simulink model "Dianlan_deng"  (R2021a)
settings: Solver=ode23tb  StartTime=0.0  StopTime=20e-6  MaxStep=0.2  RelTol=1e-4  EnableMultiTasking=on
PreLoadFcn:
  | % -- Recommended Settings --
  | %
  | %  Simulink:
  | %      Solver: Ode23tb
  | %      Relative tolerance = 1e-4
  | %      Max step size = 0.2
  | %
  | %  Powergui:
  |          Ts = 0; % (continuous electrical model)
  | %
  | %
  | % ----------------------------------
libraries: spsVoltageMeasurementLib x4, spsDistributedParametersLineLib x3, spsGroundLib x3, spsSeriesRLCBranchLib x3, spsControlledVoltageSourceLib x1, spspowerguiLib x1
settings Model: Creator=Administrator  LastModifiedBy=张瑞
settings SolverCC: AlgebraicLoopSolver=TrustRegion
settings DataIOCC: LimitDataPoints=on  ReturnWorkspaceOutputs=off
settings OptimizationCC: LifeSpan=inf
settings DebuggingCC: AllowSymbolicDim=off  SFUnexpectedBacktrackingDiag=warning  SFNoUnconditionalDefaultTransitionDiag=warning  SFMachineParentedDataDiag=warning  ArithmeticOperatorsInVariantConditions=warning
settings SFSimCC: SimUseLocalCustomCode=off  CustomCodeUndefinedFunction=UseInterfaceOnly
settings RTWCC: RTWUseLocalCustomCode=off
settings CodeAppCC: StateflowObjectComments=on
settings GRTTargetCC: TargetLangStandard=C89/C90 (ANSI)
settings ConfigComp: CovMetricSettings=dw  CovSaveCumulativeToWorkspaceVar=on  CovSaveSingleToWorkspaceVar=on  CovExternalEMLEnable=off  CovSFcnEnable=off
settings SimscapeCC: SimscapeNormalizeSystem=off

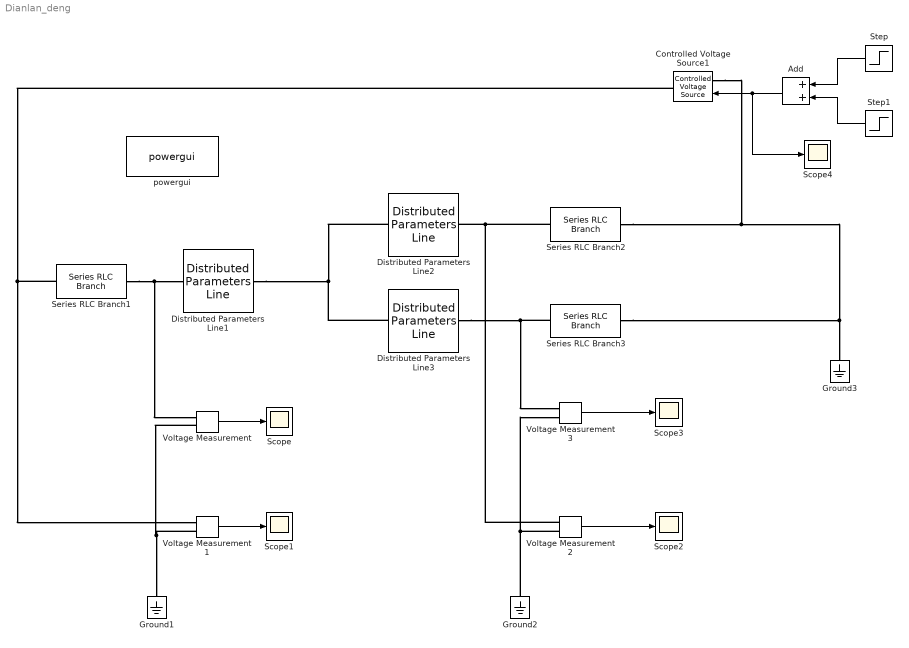
== system Dianlan_deng ==
  Add : Sum
  Controlled Voltage Source1 : spsControlledVoltageSourceLib/Controlled Voltage Source  Initialize=off  Source_Type=DC  Amplitude=0  Phase=0  Frequency=0  Measurements=Voltage
  Distributed Parameters Line1 : spsDistributedParametersLineLib/Distributed Parameters Line  Phases=1  Length=0.2  Frequency=1000  Resistance=1.8E-1  Inductance=2.75E-4  Capacitance=5.57E-7  x1=[-2.48e-06 0;-2.47e-06 0;-2.46e-06 0;-2.45e-06 0;-2.44e-06 0;-2.43e-06 0;-2.42e-06 0;-2.41e-06 0;-2.4e-06 0;-2.39e-06 0;-2.38e-06 0;-2.37e-06 0;-2.36e-06 0;-2.35e-06 0;-2.34e-06 0;-2.33e-06 0;-2.32e-06 0;-2.31e-06 0;-2.3e-06 0;-2.29e-06 0;-2.28e-06 0;-2.27e-06 0;-2.26e-06 0;-2.25e-06 0;-2.24e-06 0;-2.23e-06 0;-2.22e-06 0;-2.21e-06 0;-2.2e-06 0;-2.19e-06 0;-2.18e-06 0;-2.17e-06 0;-2.16e-06 0;-2.15e-06 0;-2.14e-06 0;-2.13e-06 0;-2.12e-06 0;-2.11e-06 0;-2.1e-06 0;-2.09e-06 0;-2.08e-06 0;-2.07e-06 0;-2.06e-06 0;-2.05e-06 0;-2.04e-06 0;-2.03e-06 0;-2.02e-06 0;-2.01e-06 0;-2e-06 0;-1.99e-06 0;-1.98e-06 0;-1.97e-06 0;-1.96e-06 0;-1.95e-06 0;-1.94e-06 0;-1.93e-06 0;-1.92e-06 0;-1.91e-06 0;-1.9e-06 0;-1.89e-06 0;-1.88e-06 0;-1.87e-06 0;-1.86e-06 0;-1.85e-06 0;-1.84e-06 0;-1.83e-06 0;-1.82e-06 0;-1.81e-06 0;-1.8e-06 0;-1.79e-06 0;-1.78e-06 0;-1.77e-06 0;-1.76e-06 0;-1.75e-06 0;-1.74e-06 0;-1.73e-06 0;-1.72e-06 0;-1.71e-06 0;-1.7e-06 0;-1.69e-06 0;-1.68e-06 0;-1.67e-06 0;-1.66e-06 0;-1.65e-06 0;-1.64e-06 0;-1.63e-06 0;-1.62e-06 0;-1.61e-06 0;-1.6e-06 0;-1.59e-06 0;-1.58e-06 0;-1.57e-06 0;-1.56e-06 0;-1.55e-06 0;-1.54e-06 0;-1.53e-06 0;-1.52e-06 0;-1.51e-06 0;-1.5e-06 0;-1.49e-06 0;-1.48e-06 0;-1.47e-06 0;-1.46e-06 0;-1.45e-06 0;-1.44e-06 0;-1.43e-06 0;-1.42e-06 0;-1.41e-06 0;-1.4e-06 0;-1.39e-06 0;-1.38e-06 0;-1.37e-06 0;-1.36e-06 0;-1.35e-06 0;-1.34e-06 0;-1.33e-06 0;-1.32e-06 0;-1.31e-06 0;-1.3e-06 0;-1.29e-06 0;-1.28e-06 0;-1.27e-06 0;-1.26e-06 0;-1.25e-06 0;-1.24e-06 0;-1.23e-06 0;-1.22e-06 0;-1.21e-06 0;-1.2e-06 0;-1.19e-06 0;-1.18e-06 0;-1.17e-06 0;-1.16e-06 0;-1.15e-06 0;-1.14e-06 0;-1.13e-06 0;-1.12e-06 0;-1.11e-06 0;-1.1e-06 0;-1.09e-06 0;-1.08e-06 0;-1.07e-06 0;-1.06e-06 0;-1.05e-06 0;-1.04e-06 0;-1.03e-06 0;-1.02e-06 0;-1.01e-06 0;-1e-06 0;-9.9e-07 0;-9.8e-07 0;-9.7e-07 0;-9.6e-07 0;-9.5e-07 0;-9.4e-07 0;-9.3e-07 0;-9.2e-07 0;-9.1e-07 0;-9e-07 0;-8.9e-07 0;-8.8e-07 0;-8.7e-07 0;-8.6e-07 0;-8.5e-07 0;-8.4e-07 0;-8.3e-07 0;-8.2e-07 0;-8.1e-07 0;-8e-07 0;-7.9e-07 0;-7.8e-07 0;-7.7e-07 0;-7.6e-07 0;-7.5e-07 0;-7.4e-07 0;-7.3e-07 0;-7.2e-07 0;-7.1e-07 0;-7e-07 0;-6.9e-07 0;-6.8e-07 0;-6.7e-07 0;-6.6e-07 0;-6.5e-07 0;-6.4e-07 0;-6.3e-07 0;-6.2e-07 0;-6.1e-07 0;-6e-07 0;-5.9e-07 0;-5.8e-07 0;-5.7e-07 0;-5.6e-07 0;-5.5e-07 0;-5.4e-07 0;-5.3e-07 0;-5.2e-07 0;-5.1e-07 0;-5e-07 0;-4.9e-07 0;-4.8e-07 0;-4.7e-07 0;-4.6e-07 0;-4.5e-07 0;-4.4e-07 0;-4.3e-07 0;-4.2e-07 0;-4.1e-07 0;-4e-07 0;-3.9e-07 0;-3.8e-07 0;-3.7e-07 0;-3.6e-07 0;-3.5e-07 0;-3.4e-07 0;-3.3e-07 0;-3.2e-07 0;-3.1e-07 0;-3e-07 0;-2.9e-07 0;-2.8e-07 0;-2.7e-07 0;-2.6e-07 0;-2.5e-07 0;-2.4e-07 0;-2.3e-07 0;-2.2e-07 0;-2.1e-07 0;-2e-07 0;-1.9e-07 0;-1.8e-07 0;-1.7e-07 0;-1.6e-07 0;-1.5e-07 0;-1.4e-07 0;-1.3e-07 0;-1.2e-07 0;-1.1e-07 0;-1e-07 0;-9e-08 0;-8e-08 0;-7e-08 0;-6e-08 0;-5e-08 0;-4e-08 0;-3e-08 0;-2e-08 0;-1e-08 0]  x2=[-2.48e-06 0;-2.47e-06 0;-2.46e-06 0;-2.45e-06 0;-2.44e-06 0;-2.43e-06 0;-2.42e-06 0;-2.41e-06 0;-2.4e-06 0;-2.39e-06 0;-2.38e-06 0;-2.37e-06 0;-2.36e-06 0;-2.35e-06 0;-2.34e-06 0;-2.33e-06 0;-2.32e-06 0;-2.31e-06 0;-2.3e-06 0;-2.29e-06 0;-2.28e-06 0;-2.27e-06 0;-2.26e-06 0;-2.25e-06 0;-2.24e-06 0;-2.23e-06 0;-2.22e-06 0;-2.21e-06 0;-2.2e-06 0;-2.19e-06 0;-2.18e-06 0;-2.17e-06 0;-2.16e-06 0;-2.15e-06 0;-2.14e-06 0;-2.13e-06 0;-2.12e-06 0;-2.11e-06 0;-2.1e-06 0;-2.09e-06 0;-2.08e-06 0;-2.07e-06 0;-2.06e-06 0;-2.05e-06 0;-2.04e-06 0;-2.03e-06 0;-2.02e-06 0;-2.01e-06 0;-2e-06 0;-1.99e-06 0;-1.98e-06 0;-1.97e-06 0;-1.96e-06 0;-1.95e-06 0;-1.94e-06 0;-1.93e-06 0;-1.92e-06 0;-1.91e-06 0;-1.9e-06 0;-1.89e-06 0;-1.88e-06 0;-1.87e-06 0;-1.86e-06 0;-1.85e-06 0;-1.84e-06 0;-1.83e-06 0;-1.82e-06 0;-1.81e-06 0;-1.8e-06 0;-1.79e-06 0;-1.78e-06 0;-1.77e-06 0;-1.76e-06 0;-1.75e-06 0;-1.74e-06 0;-1.73e-06 0;-1.72e-06 0;-1.71e-06 0;-1.7e-06 0;-1.69e-06 0;-1.68e-06 0;-1.67e-06 0;-1.66e-06 0;-1.65e-06 0;-1.64e-06 0;-1.63e-06 0;-1.62e-06 0;-1.61e-06 0;-1.6e-06 0;-1.59e-06 0;-1.58e-06 0;-1.57e-06 0;-1.56e-06 0;-1.55e-06 0;-1.54e-06 0;-1.53e-06 0;-1.52e-06 0;-1.51e-06 0;-1.5e-06 0;-1.49e-06 0;-1.48e-06 0;-1.47e-06 0;-1.46e-06 0;-1.45e-06 0;-1.44e-06 0;-1.43e-06 0;-1.42e-06 0;-1.41e-06 0;-1.4e-06 0;-1.39e-06 0;-1.38e-06 0;-1.37e-06 0;-1.36e-06 0;-1.35e-06 0;-1.34e-06 0;-1.33e-06 0;-1.32e-06 0;-1.31e-06 0;-1.3e-06 0;-1.29e-06 0;-1.28e-06 0;-1.27e-06 0;-1.26e-06 0;-1.25e-06 0;-1.24e-06 0;-1.23e-06 0;-1.22e-06 0;-1.21e-06 0;-1.2e-06 0;-1.19e-06 0;-1.18e-06 0;-1.17e-06 0;-1.16e-06 0;-1.15e-06 0;-1.14e-06 0;-1.13e-06 0;-1.12e-06 0;-1.11e-06 0;-1.1e-06 0;-1.09e-06 0;-1.08e-06 0;-1.07e-06 0;-1.06e-06 0;-1.05e-06 0;-1.04e-06 0;-1.03e-06 0;-1.02e-06 0;-1.01e-06 0;-1e-06 0;-9.9e-07 0;-9.8e-07 0;-9.7e-07 0;-9.6e-07 0;-9.5e-07 0;-9.4e-07 0;-9.3e-07 0;-9.2e-07 0;-9.1e-07 0;-9e-07 0;-8.9e-07 0;-8.8e-07 0;-8.7e-07 0;-8.6e-07 0;-8.5e-07 0;-8.4e-07 0;-8.3e-07 0;-8.2e-07 0;-8.1e-07 0;-8e-07 0;-7.9e-07 0;-7.8e-07 0;-7.7e-07 0;-7.6e-07 0;-7.5e-07 0;-7.4e-07 0;-7.3e-07 0;-7.2e-07 0;-7.1e-07 0;-7e-07 0;-6.9e-07 0;-6.8e-07 0;-6.7e-07 0;-6.6e-07 0;-6.5e-07 0;-6.4e-07 0;-6.3e-07 0;-6.2e-07 0;-6.1e-07 0;-6e-07 0;-5.9e-07 0;-5.8e-07 0;-5.7e-07 0;-5.6e-07 0;-5.5e-07 0;-5.4e-07 0;-5.3e-07 0;-5.2e-07 0;-5.1e-07 0;-5e-07 0;-4.9e-07 0;-4.8e-07 0;-4.7e-07 0;-4.6e-07 0;-4.5e-07 0;-4.4e-07 0;-4.3e-07 0;-4.2e-07 0;-4.1e-07 0;-4e-07 0;-3.9e-07 0;-3.8e-07 0;-3.7e-07 0;-3.6e-07 0;-3.5e-07 0;-3.4e-07 0;-3.3e-07 0;-3.2e-07 0;-3.1e-07 0;-3e-07 0;-2.9e-07 0;-2.8e-07 0;-2.7e-07 0;-2.6e-07 0;-2.5e-07 0;-2.4e-07 0;-2.3e-07 0;-2.2e-07 0;-2.1e-07 0;-2e-07 0;-1.9e-07 0;-1.8e-07 0;-1.7e-07 0;-1.6e-07 0;-1.5e-07 0;-1.4e-07 0;-1.3e-07 0;-1.2e-07 0;-1.1e-07 0;-1e-07 0;-9e-08 0;-8e-08 0;-7e-08 0;-6e-08 0;-5e-08 0;-4e-08 0;-3e-08 0;-2e-08 0;-1e-08 0]  x3=[-2.48e-06 0;-2.47e-06 0;-2.46e-06 0;-2.45e-06 0;-2.44e-06 0;-2.43e-06 0;-2.42e-06 0;-2.41e-06 0;-2.4e-06 0;-2.39e-06 0;-2.38e-06 0;-2.37e-06 0;-2.36e-06 0;-2.35e-06 0;-2.34e-06 0;-2.33e-06 0;-2.32e-06 0;-2.31e-06 0;-2.3e-06 0;-2.29e-06 0;-2.28e-06 0;-2.27e-06 0;-2.26e-06 0;-2.25e-06 0;-2.24e-06 0;-2.23e-06 0;-2.22e-06 0;-2.21e-06 0;-2.2e-06 0;-2.19e-06 0;-2.18e-06 0;-2.17e-06 0;-2.16e-06 0;-2.15e-06 0;-2.14e-06 0;-2.13e-06 0;-2.12e-06 0;-2.11e-06 0;-2.1e-06 0;-2.09e-06 0;-2.08e-06 0;-2.07e-06 0;-2.06e-06 0;-2.05e-06 0;-2.04e-06 0;-2.03e-06 0;-2.02e-06 0;-2.01e-06 0;-2e-06 0;-1.99e-06 0;-1.98e-06 0;-1.97e-06 0;-1.96e-06 0;-1.95e-06 0;-1.94e-06 0;-1.93e-06 0;-1.92e-06 0;-1.91e-06 0;-1.9e-06 0;-1.89e-06 0;-1.88e-06 0;-1.87e-06 0;-1.86e-06 0;-1.85e-06 0;-1.84e-06 0;-1.83e-06 0;-1.82e-06 0;-1.81e-06 0;-1.8e-06 0;-1.79e-06 0;-1.78e-06 0;-1.77e-06 0;-1.76e-06 0;-1.75e-06 0;-1.74e-06 0;-1.73e-06 0;-1.72e-06 0;-1.71e-06 0;-1.7e-06 0;-1.69e-06 0;-1.68e-06 0;-1.67e-06 0;-1.66e-06 0;-1.65e-06 0;-1.64e-06 0;-1.63e-06 0;-1.62e-06 0;-1.61e-06 0;-1.6e-06 0;-1.59e-06 0;-1.58e-06 0;-1.57e-06 0;-1.56e-06 0;-1.55e-06 0;-1.54e-06 0;-1.53e-06 0;-1.52e-06 0;-1.51e-06 0;-1.5e-06 0;-1.49e-06 0;-1.48e-06 0;-1.47e-06 0;-1.46e-06 0;-1.45e-06 0;-1.44e-06 0;-1.43e-06 0;-1.42e-06 0;-1.41e-06 0;-1.4e-06 0;-1.39e-06 0;-1.38e-06 0;-1.37e-06 0;-1.36e-06 0;-1.35e-06 0;-1.34e-06 0;-1.33e-06 0;-1.32e-06 0;-1.31e-06 0;-1.3e-06 0;-1.29e-06 0;-1.28e-06 0;-1.27e-06 0;-1.26e-06 0;-1.25e-06 0;-1.24e-06 0;-1.23e-06 0;-1.22e-06 0;-1.21e-06 0;-1.2e-06 0;-1.19e-06 0;-1.18e-06 0;-1.17e-06 0;-1.16e-06 0;-1.15e-06 0;-1.14e-06 0;-1.13e-06 0;-1.12e-06 0;-1.11e-06 0;-1.1e-06 0;-1.09e-06 0;-1.08e-06 0;-1.07e-06 0;-1.06e-06 0;-1.05e-06 0;-1.04e-06 0;-1.03e-06 0;-1.02e-06 0;-1.01e-06 0;-1e-06 0;-9.9e-07 0;-9.8e-07 0;-9.7e-07 0;-9.6e-07 0;-9.5e-07 0;-9.4e-07 0;-9.3e-07 0;-9.2e-07 0;-9.1e-07 0;-9e-07 0;-8.9e-07 0;-8.8e-07 0;-8.7e-07 0;-8.6e-07 0;-8.5e-07 0;-8.4e-07 0;-8.3e-07 0;-8.2e-07 0;-8.1e-07 0;-8e-07 0;-7.9e-07 0;-7.8e-07 0;-7.7e-07 0;-7.6e-07 0;-7.5e-07 0;-7.4e-07 0;-7.3e-07 0;-7.2e-07 0;-7.1e-07 0;-7e-07 0;-6.9e-07 0;-6.8e-07 0;-6.7e-07 0;-6.6e-07 0;-6.5e-07 0;-6.4e-07 0;-6.3e-07 0;-6.2e-07 0;-6.1e-07 0;-6e-07 0;-5.9e-07 0;-5.8e-07 0;-5.7e-07 0;-5.6e-07 0;-5.5e-07 0;-5.4e-07 0;-5.3e-07 0;-5.2e-07 0;-5.1e-07 0;-5e-07 0;-4.9e-07 0;-4.8e-07 0;-4.7e-07 0;-4.6e-07 0;-4.5e-07 0;-4.4e-07 0;-4.3e-07 0;-4.2e-07 0;-4.1e-07 0;-4e-07 0;-3.9e-07 0;-3.8e-07 0;-3.7e-07 0;-3.6e-07 0;-3.5e-07 0;-3.4e-07 0;-3.3e-07 0;-3.2e-07 0;-3.1e-07 0;-3e-07 0;-2.9e-07 0;-2.8e-07 0;-2.7e-07 0;-2.6e-07 0;-2.5e-07 0;-2.4e-07 0;-2.3e-07 0;-2.2e-07 0;-2.1e-07 0;-2e-07 0;-1.9e-07 0;-1.8e-07 0;-1.7e-07 0;-1.6e-07 0;-1.5e-07 0;-1.4e-07 0;-1.3e-07 0;-1.2e-07 0;-1.1e-07 0;-1e-07 0;-9e-08 0;-8e-08 0;-7e-08 0;-6e-08 0;-5e-08 0;-4e-08 0;-3e-08 0;-2e-08 0;-1e-08 0]  x4=[-2.48e-06 0;-2.47e-06 0;-2.46e-06 0;-2.45e-06 0;-2.44e-06 0;-2.43e-06 0;-2.42e-06 0;-2.41e-06 0;-2.4e-06 0;-2.39e-06 0;-2.38e-06 0;-2.37e-06 0;-2.36e-06 0;-2.35e-06 0;-2.34e-06 0;-2.33e-06 0;-2.32e-06 0;-2.31e-06 0;-2.3e-06 0;-2.29e-06 0;-2.28e-06 0;-2.27e-06 0;-2.26e-06 0;-2.25e-06 0;-2.24e-06 0;-2.23e-06 0;-2.22e-06 0;-2.21e-06 0;-2.2e-06 0;-2.19e-06 0;-2.18e-06 0;-2.17e-06 0;-2.16e-06 0;-2.15e-06 0;-2.14e-06 0;-2.13e-06 0;-2.12e-06 0;-2.11e-06 0;-2.1e-06 0;-2.09e-06 0;-2.08e-06 0;-2.07e-06 0;-2.06e-06 0;-2.05e-06 0;-2.04e-06 0;-2.03e-06 0;-2.02e-06 0;-2.01e-06 0;-2e-06 0;-1.99e-06 0;-1.98e-06 0;-1.97e-06 0;-1.96e-06 0;-1.95e-06 0;-1.94e-06 0;-1.93e-06 0;-1.92e-06 0;-1.91e-06 0;-1.9e-06 0;-1.89e-06 0;-1.88e-06 0;-1.87e-06 0;-1.86e-06 0;-1.85e-06 0;-1.84e-06 0;-1.83e-06 0;-1.82e-06 0;-1.81e-06 0;-1.8e-06 0;-1.79e-06 0;-1.78e-06 0;-1.77e-06 0;-1.76e-06 0;-1.75e-06 0;-1.74e-06 0;-1.73e-06 0;-1.72e-06 0;-1.71e-06 0;-1.7e-06 0;-1.69e-06 0;-1.68e-06 0;-1.67e-06 0;-1.66e-06 0;-1.65e-06 0;-1.64e-06 0;-1.63e-06 0;-1.62e-06 0;-1.61e-06 0;-1.6e-06 0;-1.59e-06 0;-1.58e-06 0;-1.57e-06 0;-1.56e-06 0;-1.55e-06 0;-1.54e-06 0;-1.53e-06 0;-1.52e-06 0;-1.51e-06 0;-1.5e-06 0;-1.49e-06 0;-1.48e-06 0;-1.47e-06 0;-1.46e-06 0;-1.45e-06 0;-1.44e-06 0;-1.43e-06 0;-1.42e-06 0;-1.41e-06 0;-1.4e-06 0;-1.39e-06 0;-1.38e-06 0;-1.37e-06 0;-1.36e-06 0;-1.35e-06 0;-1.34e-06 0;-1.33e-06 0;-1.32e-06 0;-1.31e-06 0;-1.3e-06 0;-1.29e-06 0;-1.28e-06 0;-1.27e-06 0;-1.26e-06 0;-1.25e-06 0;-1.24e-06 0;-1.23e-06 0;-1.22e-06 0;-1.21e-06 0;-1.2e-06 0;-1.19e-06 0;-1.18e-06 0;-1.17e-06 0;-1.16e-06 0;-1.15e-06 0;-1.14e-06 0;-1.13e-06 0;-1.12e-06 0;-1.11e-06 0;-1.1e-06 0;-1.09e-06 0;-1.08e-06 0;-1.07e-06 0;-1.06e-06 0;-1.05e-06 0;-1.04e-06 0;-1.03e-06 0;-1.02e-06 0;-1.01e-06 0;-1e-06 0;-9.9e-07 0;-9.8e-07 0;-9.7e-07 0;-9.6e-07 0;-9.5e-07 0;-9.4e-07 0;-9.3e-07 0;-9.2e-07 0;-9.1e-07 0;-9e-07 0;-8.9e-07 0;-8.8e-07 0;-8.7e-07 0;-8.6e-07 0;-8.5e-07 0;-8.4e-07 0;-8.3e-07 0;-8.2e-07 0;-8.1e-07 0;-8e-07 0;-7.9e-07 0;-7.8e-07 0;-7.7e-07 0;-7.6e-07 0;-7.5e-07 0;-7.4e-07 0;-7.3e-07 0;-7.2e-07 0;-7.1e-07 0;-7e-07 0;-6.9e-07 0;-6.8e-07 0;-6.7e-07 0;-6.6e-07 0;-6.5e-07 0;-6.4e-07 0;-6.3e-07 0;-6.2e-07 0;-6.1e-07 0;-6e-07 0;-5.9e-07 0;-5.8e-07 0;-5.7e-07 0;-5.6e-07 0;-5.5e-07 0;-5.4e-07 0;-5.3e-07 0;-5.2e-07 0;-5.1e-07 0;-5e-07 0;-4.9e-07 0;-4.8e-07 0;-4.7e-07 0;-4.6e-07 0;-4.5e-07 0;-4.4e-07 0;-4.3e-07 0;-4.2e-07 0;-4.1e-07 0;-4e-07 0;-3.9e-07 0;-3.8e-07 0;-3.7e-07 0;-3.6e-07 0;-3.5e-07 0;-3.4e-07 0;-3.3e-07 0;-3.2e-07 0;-3.1e-07 0;-3e-07 0;-2.9e-07 0;-2.8e-07 0;-2.7e-07 0;-2.6e-07 0;-2.5e-07 0;-2.4e-07 0;-2.3e-07 0;-2.2e-07 0;-2.1e-07 0;-2e-07 0;-1.9e-07 0;-1.8e-07 0;-1.7e-07 0;-1.6e-07 0;-1.5e-07 0;-1.4e-07 0;-1.3e-07 0;-1.2e-07 0;-1.1e-07 0;-1e-07 0;-9e-08 0;-8e-08 0;-7e-08 0;-6e-08 0;-5e-08 0;-4e-08 0;-3e-08 0;-2e-08 0;-1e-08 0]  x5=2.47527776219155e-06  V1=[0;0;1.571]  V2=[0;0;1.571]  I1=[0;0;1.571]  I2=[0;0;1.571]  nHarmo=1  Measurements=Phase-to-ground voltages  Decoupling=off  VsMag0=0  VrMag0=0  VsAngle0=0  VrAngle0=0  IsMag0=0  IrMag0=0  IsAngle0=0  IrAngle0=0
      settings: SourceProductBaseCode=PS
  Distributed Parameters Line2 : spsDistributedParametersLineLib/Distributed Parameters Line  Phases=1  Length=0.2  Frequency=1000  Resistance=1.8E-1  Inductance=2.75E-4  Capacitance=5.57E-7  x1=[-2.48e-06 0;-2.47e-06 0;-2.46e-06 0;-2.45e-06 0;-2.44e-06 0;-2.43e-06 0;-2.42e-06 0;-2.41e-06 0;-2.4e-06 0;-2.39e-06 0;-2.38e-06 0;-2.37e-06 0;-2.36e-06 0;-2.35e-06 0;-2.34e-06 0;-2.33e-06 0;-2.32e-06 0;-2.31e-06 0;-2.3e-06 0;-2.29e-06 0;-2.28e-06 0;-2.27e-06 0;-2.26e-06 0;-2.25e-06 0;-2.24e-06 0;-2.23e-06 0;-2.22e-06 0;-2.21e-06 0;-2.2e-06 0;-2.19e-06 0;-2.18e-06 0;-2.17e-06 0;-2.16e-06 0;-2.15e-06 0;-2.14e-06 0;-2.13e-06 0;-2.12e-06 0;-2.11e-06 0;-2.1e-06 0;-2.09e-06 0;-2.08e-06 0;-2.07e-06 0;-2.06e-06 0;-2.05e-06 0;-2.04e-06 0;-2.03e-06 0;-2.02e-06 0;-2.01e-06 0;-2e-06 0;-1.99e-06 0;-1.98e-06 0;-1.97e-06 0;-1.96e-06 0;-1.95e-06 0;-1.94e-06 0;-1.93e-06 0;-1.92e-06 0;-1.91e-06 0;-1.9e-06 0;-1.89e-06 0;-1.88e-06 0;-1.87e-06 0;-1.86e-06 0;-1.85e-06 0;-1.84e-06 0;-1.83e-06 0;-1.82e-06 0;-1.81e-06 0;-1.8e-06 0;-1.79e-06 0;-1.78e-06 0;-1.77e-06 0;-1.76e-06 0;-1.75e-06 0;-1.74e-06 0;-1.73e-06 0;-1.72e-06 0;-1.71e-06 0;-1.7e-06 0;-1.69e-06 0;-1.68e-06 0;-1.67e-06 0;-1.66e-06 0;-1.65e-06 0;-1.64e-06 0;-1.63e-06 0;-1.62e-06 0;-1.61e-06 0;-1.6e-06 0;-1.59e-06 0;-1.58e-06 0;-1.57e-06 0;-1.56e-06 0;-1.55e-06 0;-1.54e-06 0;-1.53e-06 0;-1.52e-06 0;-1.51e-06 0;-1.5e-06 0;-1.49e-06 0;-1.48e-06 0;-1.47e-06 0;-1.46e-06 0;-1.45e-06 0;-1.44e-06 0;-1.43e-06 0;-1.42e-06 0;-1.41e-06 0;-1.4e-06 0;-1.39e-06 0;-1.38e-06 0;-1.37e-06 0;-1.36e-06 0;-1.35e-06 0;-1.34e-06 0;-1.33e-06 0;-1.32e-06 0;-1.31e-06 0;-1.3e-06 0;-1.29e-06 0;-1.28e-06 0;-1.27e-06 0;-1.26e-06 0;-1.25e-06 0;-1.24e-06 0;-1.23e-06 0;-1.22e-06 0;-1.21e-06 0;-1.2e-06 0;-1.19e-06 0;-1.18e-06 0;-1.17e-06 0;-1.16e-06 0;-1.15e-06 0;-1.14e-06 0;-1.13e-06 0;-1.12e-06 0;-1.11e-06 0;-1.1e-06 0;-1.09e-06 0;-1.08e-06 0;-1.07e-06 0;-1.06e-06 0;-1.05e-06 0;-1.04e-06 0;-1.03e-06 0;-1.02e-06 0;-1.01e-06 0;-1e-06 0;-9.9e-07 0;-9.8e-07 0;-9.7e-07 0;-9.6e-07 0;-9.5e-07 0;-9.4e-07 0;-9.3e-07 0;-9.2e-07 0;-9.1e-07 0;-9e-07 0;-8.9e-07 0;-8.8e-07 0;-8.7e-07 0;-8.6e-07 0;-8.5e-07 0;-8.4e-07 0;-8.3e-07 0;-8.2e-07 0;-8.1e-07 0;-8e-07 0;-7.9e-07 0;-7.8e-07 0;-7.7e-07 0;-7.6e-07 0;-7.5e-07 0;-7.4e-07 0;-7.3e-07 0;-7.2e-07 0;-7.1e-07 0;-7e-07 0;-6.9e-07 0;-6.8e-07 0;-6.7e-07 0;-6.6e-07 0;-6.5e-07 0;-6.4e-07 0;-6.3e-07 0;-6.2e-07 0;-6.1e-07 0;-6e-07 0;-5.9e-07 0;-5.8e-07 0;-5.7e-07 0;-5.6e-07 0;-5.5e-07 0;-5.4e-07 0;-5.3e-07 0;-5.2e-07 0;-5.1e-07 0;-5e-07 0;-4.9e-07 0;-4.8e-07 0;-4.7e-07 0;-4.6e-07 0;-4.5e-07 0;-4.4e-07 0;-4.3e-07 0;-4.2e-07 0;-4.1e-07 0;-4e-07 0;-3.9e-07 0;-3.8e-07 0;-3.7e-07 0;-3.6e-07 0;-3.5e-07 0;-3.4e-07 0;-3.3e-07 0;-3.2e-07 0;-3.1e-07 0;-3e-07 0;-2.9e-07 0;-2.8e-07 0;-2.7e-07 0;-2.6e-07 0;-2.5e-07 0;-2.4e-07 0;-2.3e-07 0;-2.2e-07 0;-2.1e-07 0;-2e-07 0;-1.9e-07 0;-1.8e-07 0;-1.7e-07 0;-1.6e-07 0;-1.5e-07 0;-1.4e-07 0;-1.3e-07 0;-1.2e-07 0;-1.1e-07 0;-1e-07 0;-9e-08 0;-8e-08 0;-7e-08 0;-6e-08 0;-5e-08 0;-4e-08 0;-3e-08 0;-2e-08 0;-1e-08 0]  x2=[-2.48e-06 0;-2.47e-06 0;-2.46e-06 0;-2.45e-06 0;-2.44e-06 0;-2.43e-06 0;-2.42e-06 0;-2.41e-06 0;-2.4e-06 0;-2.39e-06 0;-2.38e-06 0;-2.37e-06 0;-2.36e-06 0;-2.35e-06 0;-2.34e-06 0;-2.33e-06 0;-2.32e-06 0;-2.31e-06 0;-2.3e-06 0;-2.29e-06 0;-2.28e-06 0;-2.27e-06 0;-2.26e-06 0;-2.25e-06 0;-2.24e-06 0;-2.23e-06 0;-2.22e-06 0;-2.21e-06 0;-2.2e-06 0;-2.19e-06 0;-2.18e-06 0;-2.17e-06 0;-2.16e-06 0;-2.15e-06 0;-2.14e-06 0;-2.13e-06 0;-2.12e-06 0;-2.11e-06 0;-2.1e-06 0;-2.09e-06 0;-2.08e-06 0;-2.07e-06 0;-2.06e-06 0;-2.05e-06 0;-2.04e-06 0;-2.03e-06 0;-2.02e-06 0;-2.01e-06 0;-2e-06 0;-1.99e-06 0;-1.98e-06 0;-1.97e-06 0;-1.96e-06 0;-1.95e-06 0;-1.94e-06 0;-1.93e-06 0;-1.92e-06 0;-1.91e-06 0;-1.9e-06 0;-1.89e-06 0;-1.88e-06 0;-1.87e-06 0;-1.86e-06 0;-1.85e-06 0;-1.84e-06 0;-1.83e-06 0;-1.82e-06 0;-1.81e-06 0;-1.8e-06 0;-1.79e-06 0;-1.78e-06 0;-1.77e-06 0;-1.76e-06 0;-1.75e-06 0;-1.74e-06 0;-1.73e-06 0;-1.72e-06 0;-1.71e-06 0;-1.7e-06 0;-1.69e-06 0;-1.68e-06 0;-1.67e-06 0;-1.66e-06 0;-1.65e-06 0;-1.64e-06 0;-1.63e-06 0;-1.62e-06 0;-1.61e-06 0;-1.6e-06 0;-1.59e-06 0;-1.58e-06 0;-1.57e-06 0;-1.56e-06 0;-1.55e-06 0;-1.54e-06 0;-1.53e-06 0;-1.52e-06 0;-1.51e-06 0;-1.5e-06 0;-1.49e-06 0;-1.48e-06 0;-1.47e-06 0;-1.46e-06 0;-1.45e-06 0;-1.44e-06 0;-1.43e-06 0;-1.42e-06 0;-1.41e-06 0;-1.4e-06 0;-1.39e-06 0;-1.38e-06 0;-1.37e-06 0;-1.36e-06 0;-1.35e-06 0;-1.34e-06 0;-1.33e-06 0;-1.32e-06 0;-1.31e-06 0;-1.3e-06 0;-1.29e-06 0;-1.28e-06 0;-1.27e-06 0;-1.26e-06 0;-1.25e-06 0;-1.24e-06 0;-1.23e-06 0;-1.22e-06 0;-1.21e-06 0;-1.2e-06 0;-1.19e-06 0;-1.18e-06 0;-1.17e-06 0;-1.16e-06 0;-1.15e-06 0;-1.14e-06 0;-1.13e-06 0;-1.12e-06 0;-1.11e-06 0;-1.1e-06 0;-1.09e-06 0;-1.08e-06 0;-1.07e-06 0;-1.06e-06 0;-1.05e-06 0;-1.04e-06 0;-1.03e-06 0;-1.02e-06 0;-1.01e-06 0;-1e-06 0;-9.9e-07 0;-9.8e-07 0;-9.7e-07 0;-9.6e-07 0;-9.5e-07 0;-9.4e-07 0;-9.3e-07 0;-9.2e-07 0;-9.1e-07 0;-9e-07 0;-8.9e-07 0;-8.8e-07 0;-8.7e-07 0;-8.6e-07 0;-8.5e-07 0;-8.4e-07 0;-8.3e-07 0;-8.2e-07 0;-8.1e-07 0;-8e-07 0;-7.9e-07 0;-7.8e-07 0;-7.7e-07 0;-7.6e-07 0;-7.5e-07 0;-7.4e-07 0;-7.3e-07 0;-7.2e-07 0;-7.1e-07 0;-7e-07 0;-6.9e-07 0;-6.8e-07 0;-6.7e-07 0;-6.6e-07 0;-6.5e-07 0;-6.4e-07 0;-6.3e-07 0;-6.2e-07 0;-6.1e-07 0;-6e-07 0;-5.9e-07 0;-5.8e-07 0;-5.7e-07 0;-5.6e-07 0;-5.5e-07 0;-5.4e-07 0;-5.3e-07 0;-5.2e-07 0;-5.1e-07 0;-5e-07 0;-4.9e-07 0;-4.8e-07 0;-4.7e-07 0;-4.6e-07 0;-4.5e-07 0;-4.4e-07 0;-4.3e-07 0;-4.2e-07 0;-4.1e-07 0;-4e-07 0;-3.9e-07 0;-3.8e-07 0;-3.7e-07 0;-3.6e-07 0;-3.5e-07 0;-3.4e-07 0;-3.3e-07 0;-3.2e-07 0;-3.1e-07 0;-3e-07 0;-2.9e-07 0;-2.8e-07 0;-2.7e-07 0;-2.6e-07 0;-2.5e-07 0;-2.4e-07 0;-2.3e-07 0;-2.2e-07 0;-2.1e-07 0;-2e-07 0;-1.9e-07 0;-1.8e-07 0;-1.7e-07 0;-1.6e-07 0;-1.5e-07 0;-1.4e-07 0;-1.3e-07 0;-1.2e-07 0;-1.1e-07 0;-1e-07 0;-9e-08 0;-8e-08 0;-7e-08 0;-6e-08 0;-5e-08 0;-4e-08 0;-3e-08 0;-2e-08 0;-1e-08 0]  x3=[-2.48e-06 0;-2.47e-06 0;-2.46e-06 0;-2.45e-06 0;-2.44e-06 0;-2.43e-06 0;-2.42e-06 0;-2.41e-06 0;-2.4e-06 0;-2.39e-06 0;-2.38e-06 0;-2.37e-06 0;-2.36e-06 0;-2.35e-06 0;-2.34e-06 0;-2.33e-06 0;-2.32e-06 0;-2.31e-06 0;-2.3e-06 0;-2.29e-06 0;-2.28e-06 0;-2.27e-06 0;-2.26e-06 0;-2.25e-06 0;-2.24e-06 0;-2.23e-06 0;-2.22e-06 0;-2.21e-06 0;-2.2e-06 0;-2.19e-06 0;-2.18e-06 0;-2.17e-06 0;-2.16e-06 0;-2.15e-06 0;-2.14e-06 0;-2.13e-06 0;-2.12e-06 0;-2.11e-06 0;-2.1e-06 0;-2.09e-06 0;-2.08e-06 0;-2.07e-06 0;-2.06e-06 0;-2.05e-06 0;-2.04e-06 0;-2.03e-06 0;-2.02e-06 0;-2.01e-06 0;-2e-06 0;-1.99e-06 0;-1.98e-06 0;-1.97e-06 0;-1.96e-06 0;-1.95e-06 0;-1.94e-06 0;-1.93e-06 0;-1.92e-06 0;-1.91e-06 0;-1.9e-06 0;-1.89e-06 0;-1.88e-06 0;-1.87e-06 0;-1.86e-06 0;-1.85e-06 0;-1.84e-06 0;-1.83e-06 0;-1.82e-06 0;-1.81e-06 0;-1.8e-06 0;-1.79e-06 0;-1.78e-06 0;-1.77e-06 0;-1.76e-06 0;-1.75e-06 0;-1.74e-06 0;-1.73e-06 0;-1.72e-06 0;-1.71e-06 0;-1.7e-06 0;-1.69e-06 0;-1.68e-06 0;-1.67e-06 0;-1.66e-06 0;-1.65e-06 0;-1.64e-06 0;-1.63e-06 0;-1.62e-06 0;-1.61e-06 0;-1.6e-06 0;-1.59e-06 0;-1.58e-06 0;-1.57e-06 0;-1.56e-06 0;-1.55e-06 0;-1.54e-06 0;-1.53e-06 0;-1.52e-06 0;-1.51e-06 0;-1.5e-06 0;-1.49e-06 0;-1.48e-06 0;-1.47e-06 0;-1.46e-06 0;-1.45e-06 0;-1.44e-06 0;-1.43e-06 0;-1.42e-06 0;-1.41e-06 0;-1.4e-06 0;-1.39e-06 0;-1.38e-06 0;-1.37e-06 0;-1.36e-06 0;-1.35e-06 0;-1.34e-06 0;-1.33e-06 0;-1.32e-06 0;-1.31e-06 0;-1.3e-06 0;-1.29e-06 0;-1.28e-06 0;-1.27e-06 0;-1.26e-06 0;-1.25e-06 0;-1.24e-06 0;-1.23e-06 0;-1.22e-06 0;-1.21e-06 0;-1.2e-06 0;-1.19e-06 0;-1.18e-06 0;-1.17e-06 0;-1.16e-06 0;-1.15e-06 0;-1.14e-06 0;-1.13e-06 0;-1.12e-06 0;-1.11e-06 0;-1.1e-06 0;-1.09e-06 0;-1.08e-06 0;-1.07e-06 0;-1.06e-06 0;-1.05e-06 0;-1.04e-06 0;-1.03e-06 0;-1.02e-06 0;-1.01e-06 0;-1e-06 0;-9.9e-07 0;-9.8e-07 0;-9.7e-07 0;-9.6e-07 0;-9.5e-07 0;-9.4e-07 0;-9.3e-07 0;-9.2e-07 0;-9.1e-07 0;-9e-07 0;-8.9e-07 0;-8.8e-07 0;-8.7e-07 0;-8.6e-07 0;-8.5e-07 0;-8.4e-07 0;-8.3e-07 0;-8.2e-07 0;-8.1e-07 0;-8e-07 0;-7.9e-07 0;-7.8e-07 0;-7.7e-07 0;-7.6e-07 0;-7.5e-07 0;-7.4e-07 0;-7.3e-07 0;-7.2e-07 0;-7.1e-07 0;-7e-07 0;-6.9e-07 0;-6.8e-07 0;-6.7e-07 0;-6.6e-07 0;-6.5e-07 0;-6.4e-07 0;-6.3e-07 0;-6.2e-07 0;-6.1e-07 0;-6e-07 0;-5.9e-07 0;-5.8e-07 0;-5.7e-07 0;-5.6e-07 0;-5.5e-07 0;-5.4e-07 0;-5.3e-07 0;-5.2e-07 0;-5.1e-07 0;-5e-07 0;-4.9e-07 0;-4.8e-07 0;-4.7e-07 0;-4.6e-07 0;-4.5e-07 0;-4.4e-07 0;-4.3e-07 0;-4.2e-07 0;-4.1e-07 0;-4e-07 0;-3.9e-07 0;-3.8e-07 0;-3.7e-07 0;-3.6e-07 0;-3.5e-07 0;-3.4e-07 0;-3.3e-07 0;-3.2e-07 0;-3.1e-07 0;-3e-07 0;-2.9e-07 0;-2.8e-07 0;-2.7e-07 0;-2.6e-07 0;-2.5e-07 0;-2.4e-07 0;-2.3e-07 0;-2.2e-07 0;-2.1e-07 0;-2e-07 0;-1.9e-07 0;-1.8e-07 0;-1.7e-07 0;-1.6e-07 0;-1.5e-07 0;-1.4e-07 0;-1.3e-07 0;-1.2e-07 0;-1.1e-07 0;-1e-07 0;-9e-08 0;-8e-08 0;-7e-08 0;-6e-08 0;-5e-08 0;-4e-08 0;-3e-08 0;-2e-08 0;-1e-08 0]  x4=[-2.48e-06 0;-2.47e-06 0;-2.46e-06 0;-2.45e-06 0;-2.44e-06 0;-2.43e-06 0;-2.42e-06 0;-2.41e-06 0;-2.4e-06 0;-2.39e-06 0;-2.38e-06 0;-2.37e-06 0;-2.36e-06 0;-2.35e-06 0;-2.34e-06 0;-2.33e-06 0;-2.32e-06 0;-2.31e-06 0;-2.3e-06 0;-2.29e-06 0;-2.28e-06 0;-2.27e-06 0;-2.26e-06 0;-2.25e-06 0;-2.24e-06 0;-2.23e-06 0;-2.22e-06 0;-2.21e-06 0;-2.2e-06 0;-2.19e-06 0;-2.18e-06 0;-2.17e-06 0;-2.16e-06 0;-2.15e-06 0;-2.14e-06 0;-2.13e-06 0;-2.12e-06 0;-2.11e-06 0;-2.1e-06 0;-2.09e-06 0;-2.08e-06 0;-2.07e-06 0;-2.06e-06 0;-2.05e-06 0;-2.04e-06 0;-2.03e-06 0;-2.02e-06 0;-2.01e-06 0;-2e-06 0;-1.99e-06 0;-1.98e-06 0;-1.97e-06 0;-1.96e-06 0;-1.95e-06 0;-1.94e-06 0;-1.93e-06 0;-1.92e-06 0;-1.91e-06 0;-1.9e-06 0;-1.89e-06 0;-1.88e-06 0;-1.87e-06 0;-1.86e-06 0;-1.85e-06 0;-1.84e-06 0;-1.83e-06 0;-1.82e-06 0;-1.81e-06 0;-1.8e-06 0;-1.79e-06 0;-1.78e-06 0;-1.77e-06 0;-1.76e-06 0;-1.75e-06 0;-1.74e-06 0;-1.73e-06 0;-1.72e-06 0;-1.71e-06 0;-1.7e-06 0;-1.69e-06 0;-1.68e-06 0;-1.67e-06 0;-1.66e-06 0;-1.65e-06 0;-1.64e-06 0;-1.63e-06 0;-1.62e-06 0;-1.61e-06 0;-1.6e-06 0;-1.59e-06 0;-1.58e-06 0;-1.57e-06 0;-1.56e-06 0;-1.55e-06 0;-1.54e-06 0;-1.53e-06 0;-1.52e-06 0;-1.51e-06 0;-1.5e-06 0;-1.49e-06 0;-1.48e-06 0;-1.47e-06 0;-1.46e-06 0;-1.45e-06 0;-1.44e-06 0;-1.43e-06 0;-1.42e-06 0;-1.41e-06 0;-1.4e-06 0;-1.39e-06 0;-1.38e-06 0;-1.37e-06 0;-1.36e-06 0;-1.35e-06 0;-1.34e-06 0;-1.33e-06 0;-1.32e-06 0;-1.31e-06 0;-1.3e-06 0;-1.29e-06 0;-1.28e-06 0;-1.27e-06 0;-1.26e-06 0;-1.25e-06 0;-1.24e-06 0;-1.23e-06 0;-1.22e-06 0;-1.21e-06 0;-1.2e-06 0;-1.19e-06 0;-1.18e-06 0;-1.17e-06 0;-1.16e-06 0;-1.15e-06 0;-1.14e-06 0;-1.13e-06 0;-1.12e-06 0;-1.11e-06 0;-1.1e-06 0;-1.09e-06 0;-1.08e-06 0;-1.07e-06 0;-1.06e-06 0;-1.05e-06 0;-1.04e-06 0;-1.03e-06 0;-1.02e-06 0;-1.01e-06 0;-1e-06 0;-9.9e-07 0;-9.8e-07 0;-9.7e-07 0;-9.6e-07 0;-9.5e-07 0;-9.4e-07 0;-9.3e-07 0;-9.2e-07 0;-9.1e-07 0;-9e-07 0;-8.9e-07 0;-8.8e-07 0;-8.7e-07 0;-8.6e-07 0;-8.5e-07 0;-8.4e-07 0;-8.3e-07 0;-8.2e-07 0;-8.1e-07 0;-8e-07 0;-7.9e-07 0;-7.8e-07 0;-7.7e-07 0;-7.6e-07 0;-7.5e-07 0;-7.4e-07 0;-7.3e-07 0;-7.2e-07 0;-7.1e-07 0;-7e-07 0;-6.9e-07 0;-6.8e-07 0;-6.7e-07 0;-6.6e-07 0;-6.5e-07 0;-6.4e-07 0;-6.3e-07 0;-6.2e-07 0;-6.1e-07 0;-6e-07 0;-5.9e-07 0;-5.8e-07 0;-5.7e-07 0;-5.6e-07 0;-5.5e-07 0;-5.4e-07 0;-5.3e-07 0;-5.2e-07 0;-5.1e-07 0;-5e-07 0;-4.9e-07 0;-4.8e-07 0;-4.7e-07 0;-4.6e-07 0;-4.5e-07 0;-4.4e-07 0;-4.3e-07 0;-4.2e-07 0;-4.1e-07 0;-4e-07 0;-3.9e-07 0;-3.8e-07 0;-3.7e-07 0;-3.6e-07 0;-3.5e-07 0;-3.4e-07 0;-3.3e-07 0;-3.2e-07 0;-3.1e-07 0;-3e-07 0;-2.9e-07 0;-2.8e-07 0;-2.7e-07 0;-2.6e-07 0;-2.5e-07 0;-2.4e-07 0;-2.3e-07 0;-2.2e-07 0;-2.1e-07 0;-2e-07 0;-1.9e-07 0;-1.8e-07 0;-1.7e-07 0;-1.6e-07 0;-1.5e-07 0;-1.4e-07 0;-1.3e-07 0;-1.2e-07 0;-1.1e-07 0;-1e-07 0;-9e-08 0;-8e-08 0;-7e-08 0;-6e-08 0;-5e-08 0;-4e-08 0;-3e-08 0;-2e-08 0;-1e-08 0]  x5=2.47527776219155e-06  V1=[0;0;1.571]  V2=[0;0;1.571]  I1=[0;0;1.571]  I2=[0;0;1.571]  nHarmo=1  Measurements=Phase-to-ground voltages  Decoupling=off  VsMag0=0  VrMag0=0  VsAngle0=0  VrAngle0=0  IsMag0=0  IrMag0=0  IsAngle0=0  IrAngle0=0
      settings: SourceProductBaseCode=PS
  Distributed Parameters Line3 : spsDistributedParametersLineLib/Distributed Parameters Line  Phases=1  Length=0.2  Frequency=1000  Resistance=1.8E-1  Inductance=2.75E-4  Capacitance=5.57E-7  x1=[-2.48e-06 0;-2.47e-06 0;-2.46e-06 0;-2.45e-06 0;-2.44e-06 0;-2.43e-06 0;-2.42e-06 0;-2.41e-06 0;-2.4e-06 0;-2.39e-06 0;-2.38e-06 0;-2.37e-06 0;-2.36e-06 0;-2.35e-06 0;-2.34e-06 0;-2.33e-06 0;-2.32e-06 0;-2.31e-06 0;-2.3e-06 0;-2.29e-06 0;-2.28e-06 0;-2.27e-06 0;-2.26e-06 0;-2.25e-06 0;-2.24e-06 0;-2.23e-06 0;-2.22e-06 0;-2.21e-06 0;-2.2e-06 0;-2.19e-06 0;-2.18e-06 0;-2.17e-06 0;-2.16e-06 0;-2.15e-06 0;-2.14e-06 0;-2.13e-06 0;-2.12e-06 0;-2.11e-06 0;-2.1e-06 0;-2.09e-06 0;-2.08e-06 0;-2.07e-06 0;-2.06e-06 0;-2.05e-06 0;-2.04e-06 0;-2.03e-06 0;-2.02e-06 0;-2.01e-06 0;-2e-06 0;-1.99e-06 0;-1.98e-06 0;-1.97e-06 0;-1.96e-06 0;-1.95e-06 0;-1.94e-06 0;-1.93e-06 0;-1.92e-06 0;-1.91e-06 0;-1.9e-06 0;-1.89e-06 0;-1.88e-06 0;-1.87e-06 0;-1.86e-06 0;-1.85e-06 0;-1.84e-06 0;-1.83e-06 0;-1.82e-06 0;-1.81e-06 0;-1.8e-06 0;-1.79e-06 0;-1.78e-06 0;-1.77e-06 0;-1.76e-06 0;-1.75e-06 0;-1.74e-06 0;-1.73e-06 0;-1.72e-06 0;-1.71e-06 0;-1.7e-06 0;-1.69e-06 0;-1.68e-06 0;-1.67e-06 0;-1.66e-06 0;-1.65e-06 0;-1.64e-06 0;-1.63e-06 0;-1.62e-06 0;-1.61e-06 0;-1.6e-06 0;-1.59e-06 0;-1.58e-06 0;-1.57e-06 0;-1.56e-06 0;-1.55e-06 0;-1.54e-06 0;-1.53e-06 0;-1.52e-06 0;-1.51e-06 0;-1.5e-06 0;-1.49e-06 0;-1.48e-06 0;-1.47e-06 0;-1.46e-06 0;-1.45e-06 0;-1.44e-06 0;-1.43e-06 0;-1.42e-06 0;-1.41e-06 0;-1.4e-06 0;-1.39e-06 0;-1.38e-06 0;-1.37e-06 0;-1.36e-06 0;-1.35e-06 0;-1.34e-06 0;-1.33e-06 0;-1.32e-06 0;-1.31e-06 0;-1.3e-06 0;-1.29e-06 0;-1.28e-06 0;-1.27e-06 0;-1.26e-06 0;-1.25e-06 0;-1.24e-06 0;-1.23e-06 0;-1.22e-06 0;-1.21e-06 0;-1.2e-06 0;-1.19e-06 0;-1.18e-06 0;-1.17e-06 0;-1.16e-06 0;-1.15e-06 0;-1.14e-06 0;-1.13e-06 0;-1.12e-06 0;-1.11e-06 0;-1.1e-06 0;-1.09e-06 0;-1.08e-06 0;-1.07e-06 0;-1.06e-06 0;-1.05e-06 0;-1.04e-06 0;-1.03e-06 0;-1.02e-06 0;-1.01e-06 0;-1e-06 0;-9.9e-07 0;-9.8e-07 0;-9.7e-07 0;-9.6e-07 0;-9.5e-07 0;-9.4e-07 0;-9.3e-07 0;-9.2e-07 0;-9.1e-07 0;-9e-07 0;-8.9e-07 0;-8.8e-07 0;-8.7e-07 0;-8.6e-07 0;-8.5e-07 0;-8.4e-07 0;-8.3e-07 0;-8.2e-07 0;-8.1e-07 0;-8e-07 0;-7.9e-07 0;-7.8e-07 0;-7.7e-07 0;-7.6e-07 0;-7.5e-07 0;-7.4e-07 0;-7.3e-07 0;-7.2e-07 0;-7.1e-07 0;-7e-07 0;-6.9e-07 0;-6.8e-07 0;-6.7e-07 0;-6.6e-07 0;-6.5e-07 0;-6.4e-07 0;-6.3e-07 0;-6.2e-07 0;-6.1e-07 0;-6e-07 0;-5.9e-07 0;-5.8e-07 0;-5.7e-07 0;-5.6e-07 0;-5.5e-07 0;-5.4e-07 0;-5.3e-07 0;-5.2e-07 0;-5.1e-07 0;-5e-07 0;-4.9e-07 0;-4.8e-07 0;-4.7e-07 0;-4.6e-07 0;-4.5e-07 0;-4.4e-07 0;-4.3e-07 0;-4.2e-07 0;-4.1e-07 0;-4e-07 0;-3.9e-07 0;-3.8e-07 0;-3.7e-07 0;-3.6e-07 0;-3.5e-07 0;-3.4e-07 0;-3.3e-07 0;-3.2e-07 0;-3.1e-07 0;-3e-07 0;-2.9e-07 0;-2.8e-07 0;-2.7e-07 0;-2.6e-07 0;-2.5e-07 0;-2.4e-07 0;-2.3e-07 0;-2.2e-07 0;-2.1e-07 0;-2e-07 0;-1.9e-07 0;-1.8e-07 0;-1.7e-07 0;-1.6e-07 0;-1.5e-07 0;-1.4e-07 0;-1.3e-07 0;-1.2e-07 0;-1.1e-07 0;-1e-07 0;-9e-08 0;-8e-08 0;-7e-08 0;-6e-08 0;-5e-08 0;-4e-08 0;-3e-08 0;-2e-08 0;-1e-08 0]  x2=[-2.48e-06 0;-2.47e-06 0;-2.46e-06 0;-2.45e-06 0;-2.44e-06 0;-2.43e-06 0;-2.42e-06 0;-2.41e-06 0;-2.4e-06 0;-2.39e-06 0;-2.38e-06 0;-2.37e-06 0;-2.36e-06 0;-2.35e-06 0;-2.34e-06 0;-2.33e-06 0;-2.32e-06 0;-2.31e-06 0;-2.3e-06 0;-2.29e-06 0;-2.28e-06 0;-2.27e-06 0;-2.26e-06 0;-2.25e-06 0;-2.24e-06 0;-2.23e-06 0;-2.22e-06 0;-2.21e-06 0;-2.2e-06 0;-2.19e-06 0;-2.18e-06 0;-2.17e-06 0;-2.16e-06 0;-2.15e-06 0;-2.14e-06 0;-2.13e-06 0;-2.12e-06 0;-2.11e-06 0;-2.1e-06 0;-2.09e-06 0;-2.08e-06 0;-2.07e-06 0;-2.06e-06 0;-2.05e-06 0;-2.04e-06 0;-2.03e-06 0;-2.02e-06 0;-2.01e-06 0;-2e-06 0;-1.99e-06 0;-1.98e-06 0;-1.97e-06 0;-1.96e-06 0;-1.95e-06 0;-1.94e-06 0;-1.93e-06 0;-1.92e-06 0;-1.91e-06 0;-1.9e-06 0;-1.89e-06 0;-1.88e-06 0;-1.87e-06 0;-1.86e-06 0;-1.85e-06 0;-1.84e-06 0;-1.83e-06 0;-1.82e-06 0;-1.81e-06 0;-1.8e-06 0;-1.79e-06 0;-1.78e-06 0;-1.77e-06 0;-1.76e-06 0;-1.75e-06 0;-1.74e-06 0;-1.73e-06 0;-1.72e-06 0;-1.71e-06 0;-1.7e-06 0;-1.69e-06 0;-1.68e-06 0;-1.67e-06 0;-1.66e-06 0;-1.65e-06 0;-1.64e-06 0;-1.63e-06 0;-1.62e-06 0;-1.61e-06 0;-1.6e-06 0;-1.59e-06 0;-1.58e-06 0;-1.57e-06 0;-1.56e-06 0;-1.55e-06 0;-1.54e-06 0;-1.53e-06 0;-1.52e-06 0;-1.51e-06 0;-1.5e-06 0;-1.49e-06 0;-1.48e-06 0;-1.47e-06 0;-1.46e-06 0;-1.45e-06 0;-1.44e-06 0;-1.43e-06 0;-1.42e-06 0;-1.41e-06 0;-1.4e-06 0;-1.39e-06 0;-1.38e-06 0;-1.37e-06 0;-1.36e-06 0;-1.35e-06 0;-1.34e-06 0;-1.33e-06 0;-1.32e-06 0;-1.31e-06 0;-1.3e-06 0;-1.29e-06 0;-1.28e-06 0;-1.27e-06 0;-1.26e-06 0;-1.25e-06 0;-1.24e-06 0;-1.23e-06 0;-1.22e-06 0;-1.21e-06 0;-1.2e-06 0;-1.19e-06 0;-1.18e-06 0;-1.17e-06 0;-1.16e-06 0;-1.15e-06 0;-1.14e-06 0;-1.13e-06 0;-1.12e-06 0;-1.11e-06 0;-1.1e-06 0;-1.09e-06 0;-1.08e-06 0;-1.07e-06 0;-1.06e-06 0;-1.05e-06 0;-1.04e-06 0;-1.03e-06 0;-1.02e-06 0;-1.01e-06 0;-1e-06 0;-9.9e-07 0;-9.8e-07 0;-9.7e-07 0;-9.6e-07 0;-9.5e-07 0;-9.4e-07 0;-9.3e-07 0;-9.2e-07 0;-9.1e-07 0;-9e-07 0;-8.9e-07 0;-8.8e-07 0;-8.7e-07 0;-8.6e-07 0;-8.5e-07 0;-8.4e-07 0;-8.3e-07 0;-8.2e-07 0;-8.1e-07 0;-8e-07 0;-7.9e-07 0;-7.8e-07 0;-7.7e-07 0;-7.6e-07 0;-7.5e-07 0;-7.4e-07 0;-7.3e-07 0;-7.2e-07 0;-7.1e-07 0;-7e-07 0;-6.9e-07 0;-6.8e-07 0;-6.7e-07 0;-6.6e-07 0;-6.5e-07 0;-6.4e-07 0;-6.3e-07 0;-6.2e-07 0;-6.1e-07 0;-6e-07 0;-5.9e-07 0;-5.8e-07 0;-5.7e-07 0;-5.6e-07 0;-5.5e-07 0;-5.4e-07 0;-5.3e-07 0;-5.2e-07 0;-5.1e-07 0;-5e-07 0;-4.9e-07 0;-4.8e-07 0;-4.7e-07 0;-4.6e-07 0;-4.5e-07 0;-4.4e-07 0;-4.3e-07 0;-4.2e-07 0;-4.1e-07 0;-4e-07 0;-3.9e-07 0;-3.8e-07 0;-3.7e-07 0;-3.6e-07 0;-3.5e-07 0;-3.4e-07 0;-3.3e-07 0;-3.2e-07 0;-3.1e-07 0;-3e-07 0;-2.9e-07 0;-2.8e-07 0;-2.7e-07 0;-2.6e-07 0;-2.5e-07 0;-2.4e-07 0;-2.3e-07 0;-2.2e-07 0;-2.1e-07 0;-2e-07 0;-1.9e-07 0;-1.8e-07 0;-1.7e-07 0;-1.6e-07 0;-1.5e-07 0;-1.4e-07 0;-1.3e-07 0;-1.2e-07 0;-1.1e-07 0;-1e-07 0;-9e-08 0;-8e-08 0;-7e-08 0;-6e-08 0;-5e-08 0;-4e-08 0;-3e-08 0;-2e-08 0;-1e-08 0]  x3=[-2.48e-06 0;-2.47e-06 0;-2.46e-06 0;-2.45e-06 0;-2.44e-06 0;-2.43e-06 0;-2.42e-06 0;-2.41e-06 0;-2.4e-06 0;-2.39e-06 0;-2.38e-06 0;-2.37e-06 0;-2.36e-06 0;-2.35e-06 0;-2.34e-06 0;-2.33e-06 0;-2.32e-06 0;-2.31e-06 0;-2.3e-06 0;-2.29e-06 0;-2.28e-06 0;-2.27e-06 0;-2.26e-06 0;-2.25e-06 0;-2.24e-06 0;-2.23e-06 0;-2.22e-06 0;-2.21e-06 0;-2.2e-06 0;-2.19e-06 0;-2.18e-06 0;-2.17e-06 0;-2.16e-06 0;-2.15e-06 0;-2.14e-06 0;-2.13e-06 0;-2.12e-06 0;-2.11e-06 0;-2.1e-06 0;-2.09e-06 0;-2.08e-06 0;-2.07e-06 0;-2.06e-06 0;-2.05e-06 0;-2.04e-06 0;-2.03e-06 0;-2.02e-06 0;-2.01e-06 0;-2e-06 0;-1.99e-06 0;-1.98e-06 0;-1.97e-06 0;-1.96e-06 0;-1.95e-06 0;-1.94e-06 0;-1.93e-06 0;-1.92e-06 0;-1.91e-06 0;-1.9e-06 0;-1.89e-06 0;-1.88e-06 0;-1.87e-06 0;-1.86e-06 0;-1.85e-06 0;-1.84e-06 0;-1.83e-06 0;-1.82e-06 0;-1.81e-06 0;-1.8e-06 0;-1.79e-06 0;-1.78e-06 0;-1.77e-06 0;-1.76e-06 0;-1.75e-06 0;-1.74e-06 0;-1.73e-06 0;-1.72e-06 0;-1.71e-06 0;-1.7e-06 0;-1.69e-06 0;-1.68e-06 0;-1.67e-06 0;-1.66e-06 0;-1.65e-06 0;-1.64e-06 0;-1.63e-06 0;-1.62e-06 0;-1.61e-06 0;-1.6e-06 0;-1.59e-06 0;-1.58e-06 0;-1.57e-06 0;-1.56e-06 0;-1.55e-06 0;-1.54e-06 0;-1.53e-06 0;-1.52e-06 0;-1.51e-06 0;-1.5e-06 0;-1.49e-06 0;-1.48e-06 0;-1.47e-06 0;-1.46e-06 0;-1.45e-06 0;-1.44e-06 0;-1.43e-06 0;-1.42e-06 0;-1.41e-06 0;-1.4e-06 0;-1.39e-06 0;-1.38e-06 0;-1.37e-06 0;-1.36e-06 0;-1.35e-06 0;-1.34e-06 0;-1.33e-06 0;-1.32e-06 0;-1.31e-06 0;-1.3e-06 0;-1.29e-06 0;-1.28e-06 0;-1.27e-06 0;-1.26e-06 0;-1.25e-06 0;-1.24e-06 0;-1.23e-06 0;-1.22e-06 0;-1.21e-06 0;-1.2e-06 0;-1.19e-06 0;-1.18e-06 0;-1.17e-06 0;-1.16e-06 0;-1.15e-06 0;-1.14e-06 0;-1.13e-06 0;-1.12e-06 0;-1.11e-06 0;-1.1e-06 0;-1.09e-06 0;-1.08e-06 0;-1.07e-06 0;-1.06e-06 0;-1.05e-06 0;-1.04e-06 0;-1.03e-06 0;-1.02e-06 0;-1.01e-06 0;-1e-06 0;-9.9e-07 0;-9.8e-07 0;-9.7e-07 0;-9.6e-07 0;-9.5e-07 0;-9.4e-07 0;-9.3e-07 0;-9.2e-07 0;-9.1e-07 0;-9e-07 0;-8.9e-07 0;-8.8e-07 0;-8.7e-07 0;-8.6e-07 0;-8.5e-07 0;-8.4e-07 0;-8.3e-07 0;-8.2e-07 0;-8.1e-07 0;-8e-07 0;-7.9e-07 0;-7.8e-07 0;-7.7e-07 0;-7.6e-07 0;-7.5e-07 0;-7.4e-07 0;-7.3e-07 0;-7.2e-07 0;-7.1e-07 0;-7e-07 0;-6.9e-07 0;-6.8e-07 0;-6.7e-07 0;-6.6e-07 0;-6.5e-07 0;-6.4e-07 0;-6.3e-07 0;-6.2e-07 0;-6.1e-07 0;-6e-07 0;-5.9e-07 0;-5.8e-07 0;-5.7e-07 0;-5.6e-07 0;-5.5e-07 0;-5.4e-07 0;-5.3e-07 0;-5.2e-07 0;-5.1e-07 0;-5e-07 0;-4.9e-07 0;-4.8e-07 0;-4.7e-07 0;-4.6e-07 0;-4.5e-07 0;-4.4e-07 0;-4.3e-07 0;-4.2e-07 0;-4.1e-07 0;-4e-07 0;-3.9e-07 0;-3.8e-07 0;-3.7e-07 0;-3.6e-07 0;-3.5e-07 0;-3.4e-07 0;-3.3e-07 0;-3.2e-07 0;-3.1e-07 0;-3e-07 0;-2.9e-07 0;-2.8e-07 0;-2.7e-07 0;-2.6e-07 0;-2.5e-07 0;-2.4e-07 0;-2.3e-07 0;-2.2e-07 0;-2.1e-07 0;-2e-07 0;-1.9e-07 0;-1.8e-07 0;-1.7e-07 0;-1.6e-07 0;-1.5e-07 0;-1.4e-07 0;-1.3e-07 0;-1.2e-07 0;-1.1e-07 0;-1e-07 0;-9e-08 0;-8e-08 0;-7e-08 0;-6e-08 0;-5e-08 0;-4e-08 0;-3e-08 0;-2e-08 0;-1e-08 0]  x4=[-2.48e-06 0;-2.47e-06 0;-2.46e-06 0;-2.45e-06 0;-2.44e-06 0;-2.43e-06 0;-2.42e-06 0;-2.41e-06 0;-2.4e-06 0;-2.39e-06 0;-2.38e-06 0;-2.37e-06 0;-2.36e-06 0;-2.35e-06 0;-2.34e-06 0;-2.33e-06 0;-2.32e-06 0;-2.31e-06 0;-2.3e-06 0;-2.29e-06 0;-2.28e-06 0;-2.27e-06 0;-2.26e-06 0;-2.25e-06 0;-2.24e-06 0;-2.23e-06 0;-2.22e-06 0;-2.21e-06 0;-2.2e-06 0;-2.19e-06 0;-2.18e-06 0;-2.17e-06 0;-2.16e-06 0;-2.15e-06 0;-2.14e-06 0;-2.13e-06 0;-2.12e-06 0;-2.11e-06 0;-2.1e-06 0;-2.09e-06 0;-2.08e-06 0;-2.07e-06 0;-2.06e-06 0;-2.05e-06 0;-2.04e-06 0;-2.03e-06 0;-2.02e-06 0;-2.01e-06 0;-2e-06 0;-1.99e-06 0;-1.98e-06 0;-1.97e-06 0;-1.96e-06 0;-1.95e-06 0;-1.94e-06 0;-1.93e-06 0;-1.92e-06 0;-1.91e-06 0;-1.9e-06 0;-1.89e-06 0;-1.88e-06 0;-1.87e-06 0;-1.86e-06 0;-1.85e-06 0;-1.84e-06 0;-1.83e-06 0;-1.82e-06 0;-1.81e-06 0;-1.8e-06 0;-1.79e-06 0;-1.78e-06 0;-1.77e-06 0;-1.76e-06 0;-1.75e-06 0;-1.74e-06 0;-1.73e-06 0;-1.72e-06 0;-1.71e-06 0;-1.7e-06 0;-1.69e-06 0;-1.68e-06 0;-1.67e-06 0;-1.66e-06 0;-1.65e-06 0;-1.64e-06 0;-1.63e-06 0;-1.62e-06 0;-1.61e-06 0;-1.6e-06 0;-1.59e-06 0;-1.58e-06 0;-1.57e-06 0;-1.56e-06 0;-1.55e-06 0;-1.54e-06 0;-1.53e-06 0;-1.52e-06 0;-1.51e-06 0;-1.5e-06 0;-1.49e-06 0;-1.48e-06 0;-1.47e-06 0;-1.46e-06 0;-1.45e-06 0;-1.44e-06 0;-1.43e-06 0;-1.42e-06 0;-1.41e-06 0;-1.4e-06 0;-1.39e-06 0;-1.38e-06 0;-1.37e-06 0;-1.36e-06 0;-1.35e-06 0;-1.34e-06 0;-1.33e-06 0;-1.32e-06 0;-1.31e-06 0;-1.3e-06 0;-1.29e-06 0;-1.28e-06 0;-1.27e-06 0;-1.26e-06 0;-1.25e-06 0;-1.24e-06 0;-1.23e-06 0;-1.22e-06 0;-1.21e-06 0;-1.2e-06 0;-1.19e-06 0;-1.18e-06 0;-1.17e-06 0;-1.16e-06 0;-1.15e-06 0;-1.14e-06 0;-1.13e-06 0;-1.12e-06 0;-1.11e-06 0;-1.1e-06 0;-1.09e-06 0;-1.08e-06 0;-1.07e-06 0;-1.06e-06 0;-1.05e-06 0;-1.04e-06 0;-1.03e-06 0;-1.02e-06 0;-1.01e-06 0;-1e-06 0;-9.9e-07 0;-9.8e-07 0;-9.7e-07 0;-9.6e-07 0;-9.5e-07 0;-9.4e-07 0;-9.3e-07 0;-9.2e-07 0;-9.1e-07 0;-9e-07 0;-8.9e-07 0;-8.8e-07 0;-8.7e-07 0;-8.6e-07 0;-8.5e-07 0;-8.4e-07 0;-8.3e-07 0;-8.2e-07 0;-8.1e-07 0;-8e-07 0;-7.9e-07 0;-7.8e-07 0;-7.7e-07 0;-7.6e-07 0;-7.5e-07 0;-7.4e-07 0;-7.3e-07 0;-7.2e-07 0;-7.1e-07 0;-7e-07 0;-6.9e-07 0;-6.8e-07 0;-6.7e-07 0;-6.6e-07 0;-6.5e-07 0;-6.4e-07 0;-6.3e-07 0;-6.2e-07 0;-6.1e-07 0;-6e-07 0;-5.9e-07 0;-5.8e-07 0;-5.7e-07 0;-5.6e-07 0;-5.5e-07 0;-5.4e-07 0;-5.3e-07 0;-5.2e-07 0;-5.1e-07 0;-5e-07 0;-4.9e-07 0;-4.8e-07 0;-4.7e-07 0;-4.6e-07 0;-4.5e-07 0;-4.4e-07 0;-4.3e-07 0;-4.2e-07 0;-4.1e-07 0;-4e-07 0;-3.9e-07 0;-3.8e-07 0;-3.7e-07 0;-3.6e-07 0;-3.5e-07 0;-3.4e-07 0;-3.3e-07 0;-3.2e-07 0;-3.1e-07 0;-3e-07 0;-2.9e-07 0;-2.8e-07 0;-2.7e-07 0;-2.6e-07 0;-2.5e-07 0;-2.4e-07 0;-2.3e-07 0;-2.2e-07 0;-2.1e-07 0;-2e-07 0;-1.9e-07 0;-1.8e-07 0;-1.7e-07 0;-1.6e-07 0;-1.5e-07 0;-1.4e-07 0;-1.3e-07 0;-1.2e-07 0;-1.1e-07 0;-1e-07 0;-9e-08 0;-8e-08 0;-7e-08 0;-6e-08 0;-5e-08 0;-4e-08 0;-3e-08 0;-2e-08 0;-1e-08 0]  x5=2.47527776219155e-06  V1=[0;0;1.571]  V2=[0;0;1.571]  I1=[0;0;1.571]  I2=[0;0;1.571]  nHarmo=1  Measurements=Phase-to-ground voltages  Decoupling=off  VsMag0=0  VrMag0=0  VsAngle0=0  VrAngle0=0  IsMag0=0  IrMag0=0  IsAngle0=0  IrAngle0=0
      settings: SourceProductBaseCode=PS
  Ground1 : spsGroundLib/Ground  LConnTagsString=a
  Ground2 : spsGroundLib/Ground  LConnTagsString=a
  Ground3 : spsGroundLib/Ground  LConnTagsString=a
  Scope{,1..4} (5 alike) : Scope
  Series RLC Branch1 : spsSeriesRLCBranchLib/Series RLC Branch  LConnTagsString=__new0  RConnTagsString=__new0  BranchType=R  Resistance=1  Inductance=1e-3  SetiL0=off  InitialCurrent=0  Capacitance=1e-6  Setx0=off  InitialVoltage=0  Measurements=None
  Series RLC Branch2 : spsSeriesRLCBranchLib/Series RLC Branch  LConnTagsString=__new0  RConnTagsString=__new0  BranchType=R  Resistance=0.001  Inductance=1e-3  SetiL0=off  InitialCurrent=0  Capacitance=1e-6  Setx0=off  InitialVoltage=0  Measurements=Branch voltage
  Series RLC Branch3 : spsSeriesRLCBranchLib/Series RLC Branch  LConnTagsString=__new0  RConnTagsString=__new0  BranchType=R  Resistance=0.001  Inductance=1e-3  SetiL0=off  InitialCurrent=0  Capacitance=1e-6  Setx0=off  InitialVoltage=0  Measurements=Branch voltage
  Step : Step  Time=0.3E-6  Before=28  After=0  SampleTime=1E-08
  Step1 : Step  Time=0.1E-6  Before=-28  After=0  SampleTime=1E-08
  Voltage Measurement{,1..3} (4 alike) : spsVoltageMeasurementLib/Voltage Measurement  PhasorSimulation=off  OutputType=Complex  PSBequivalent=0
  powergui : spspowerguiLib/powergui  Priority=1  SimulationMode=Discrete  SampleTime=0.01e-6  frequency=60  Iterations=50  frequencyindice=0  Pbase=100e6  ErrMax=1e-4  UnitsV=V  UnitsW=W  buscounter=0  FunctionMessages=off  echomessages=off  EnableUseOfTLC=off  CurrentSourceSwitches=off  DisableSnubberDevices=off  DisableRonSwitches=off  DisableVfSwitches=off  DisplayEquations=off  AutomaticDiscreteSolvers=off  SolverType=Tustin/Backward Euler (TBE)  Interpol=off  ExternalGateDelay=off  methode=off  Ts=100  x0status=blocks  SPID=off  SwTol=0  HookPort=off  NonlinearTolerance=1e-4  nMaxIteration=100  ContinueOnMaxIteration=off  RestoreLinks=warning  ResistiveCurrentMeasurement=off  Frange=[0:2:500]  Ylog=off  Xlog=on  ShowGrid=off  save=off  variable=ZData  structure=0  ZoomFFT=off  StartTime=0.0  cycles=1  DisplayStyle=1  fundamental=60  FreqAxis=off  MaxFrequency=1000  frequencyindicesteady=1  RmsSteady=1  display=off
  wires:
  Voltage Measurement/1 -> Scope/1
  Voltage Measurement1/1 -> Scope1/1
  Step/1 -> Add/1
  Step1/1 -> Add/2
  Add/1 -> Scope4/1, Controlled Voltage Source1/1
  Voltage Measurement3/1 -> Scope3/1
  Voltage Measurement2/1 -> Scope2/1
  connections:
  Distributed Parameters Line2/LConn1 -- Distributed Parameters Line3/LConn1 -- Distributed Parameters Line1/RConn1
  Voltage Measurement/LConn2 -- Voltage Measurement1/LConn2 -- Ground1/LConn1
  Series RLC Branch3/LConn1 -- Voltage Measurement3/LConn1 -- Distributed Parameters Line3/RConn1
  Controlled Voltage Source1/RConn1 -- Voltage Measurement1/LConn1 -- Series RLC Branch1/LConn1
  Ground2/LConn1 -- Voltage Measurement2/LConn2 -- Voltage Measurement3/LConn2
  Series RLC Branch2/RConn1 -- Controlled Voltage Source1/LConn1 -- Series RLC Branch3/RConn1 -- Ground3/LConn1
  Series RLC Branch2/LConn1 -- Voltage Measurement2/LConn1 -- Distributed Parameters Line2/RConn1
  Series RLC Branch1/RConn1 -- Voltage Measurement/LConn1 -- Distributed Parameters Line1/LConn1
